simulink model "SolarPanelVarified"  (Simulink 7.5)
settings: Solver=ode45  StartTime=0.0  StopTime=10  RelTol=1e-3
undefined symbols (not defined in the file): Hydride, Metal, Nickel
libraries: elec_lib x72, fl_lib x4, nesl_utility x4, electricdrivelib x1, powerlib x1
settings Model: Creator=Satendra  LastModifiedBy=Satendra

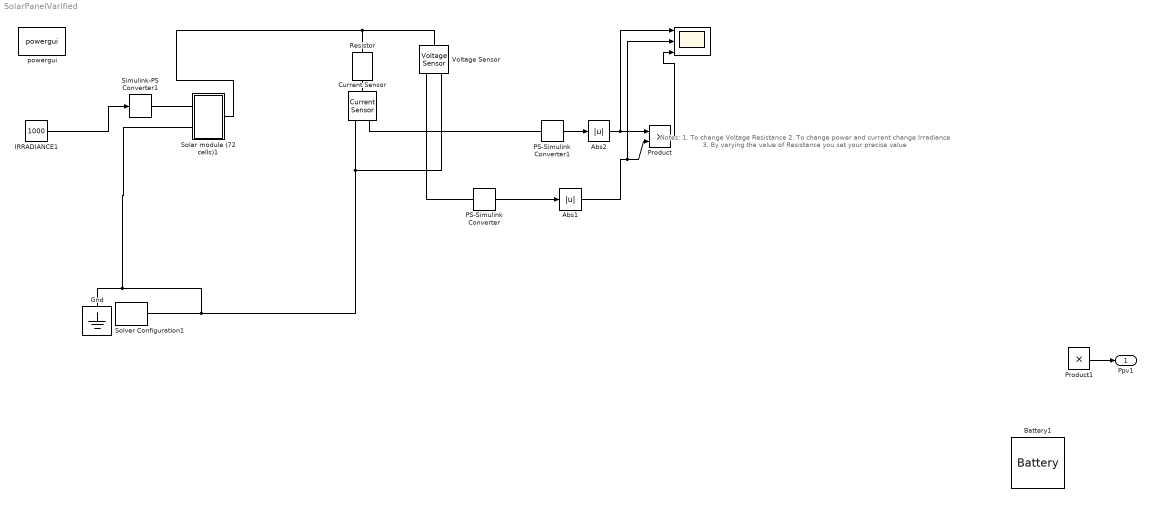
== system SolarPanelVarified ==
  note: Notes:
      | 1. To change Voltage Resistance
      | 2. To change power and current change Irradiance
      | 3. By varying the value of Resistance you set your precise value
  " " : Scope  NumInputPorts=3
      settings: TickLabels=on  YMin=-5~-5~-5  YMax=5~5~5
  Abs1 : Abs
  Abs2 : Abs
  Battery1 : electricdrivelib/Extra Sources/Battery  DialogController=POWERSYS.PowerSysDialog  SystemSampleTime=-1  BatType=Nickel-Metal-Hydride  ShowDetailedParameters=off  NomV=1.2  NomQ=1.5  SOC=100  PresetModel=on  MaxQ=1.6154  FullV=1.4136  Dis_rate=0.3  R=0.008  Normal_OP=1.4423  expZone="[1.3017         0.3]"  Dis_Char=off  current=[1.5 3]  Units=Ampere-hour  Batt_Tr=30
  Current Sensor : fl_lib/Electrical/Electrical Sensors/Current Sensor  DialogController=NetworkEngine.DynNeDlgSource  SystemSampleTime=-1  i1_Log=off  v1_Log=off  LocalVarNames=|i1|v1  LocalVarDescs=|i1|v1  LocalVarLogging=[0 0]
  Gnd : fl_lib/Electrical/Electrical Elements/Electrical Reference  DialogController=NetworkEngine.DynNeDlgSource  SystemSampleTime=-1  i_Log=off  LocalVarNames=|i  LocalVarDescs=|i  LocalVarLogging=[]
  IRRADIANCE1 : Constant  Value=1000
  PS-Simulink Converter : nesl_utility/PS-Simulink Converter  DialogController=NetworkEngine.DynNeUtilDlgSource  SystemSampleTime=-1  PhysicalDomain=network_engine_domain  LeftPortType=input  RightPortType=output  SubClassName=ps_output  Unit=1  AffineConversion=off
  PS-Simulink Converter1 : nesl_utility/PS-Simulink Converter  DialogController=NetworkEngine.DynNeUtilDlgSource  SystemSampleTime=-1  PhysicalDomain=network_engine_domain  LeftPortType=input  RightPortType=output  SubClassName=ps_output  Unit=1  AffineConversion=off
  Product : Product  RndMeth=Zero
  Product1 : Product  RndMeth=Zero
  Resistor : fl_lib/Electrical/Electrical Elements/Resistor  DialogController=NetworkEngine.DynNeDlgSource  SystemSampleTime=-1  R=3 Ohm  i_Log=off  v_Log=off  LocalVarNames=|i|v  LocalVarDescs=|i|v  LocalVarLogging=[0 0]
  Simulink-PS Converter1 : nesl_utility/Simulink-PS Converter  DialogController=NetworkEngine.DynNeUtilDlgSource  SystemSampleTime=-1  PhysicalDomain=network_engine_domain  LeftPortType=input  RightPortType=output  SubClassName=ps_input  Unit=1  AffineConversion=off  InputFilterTimeConstant=.001  UdotUserProvided=0
  Solar module (72 cells)1 : Subsystem
  Solver Configuration1 : nesl_utility/Solver Configuration  DialogController=NetworkEngine.DynNeUtilDlgSource  SystemSampleTime=-1  PhysicalDomain=network_engine_domain  LeftPortType=input  RightPortType=generic  SubClassName=solver  Accelerate=off  Profile=off  ResidualTolerance=1e-9  MaxNonlinIter=3  MaxModeIter=2  DoFixedCost=off  UseLocalSampling=off  DoDC=off  LinearAlgebra=Sparse  LocalSolverSampleTime=.001  LocalSolverChoice=NE_BACKWARD_EULER_ADVANCER  UseLocalSolver=off
  Voltage Sensor : fl_lib/Electrical/Electrical Sensors/Voltage Sensor  DialogController=NetworkEngine.DynNeDlgSource  SystemSampleTime=-1  i1_Log=off  v1_Log=off  LocalVarNames=|i1|v1  LocalVarDescs=|i1|v1  LocalVarLogging=[0 0]
  powergui : powerlib/powergui  Priority=1  SystemSampleTime=-1  SimulationMode=Continuous  SampleTime=50e-6  frequency=60  SPID=off  DisableSnubberDevices=off  DisableRonSwitches=off  DisableVfSwitches=off  SwTol=0  Interpol=off  frequencyindice=0  echomessages=off  HookPort=off  DisplayEquations=off  FunctionMessages=off  EnableUseOfTLC=off  x0status=blocks  RestoreLinks=warning  ResistiveCurrentMeasurement=off  Ylog=off  Xlog=on  ShowGrid=off  save=off  variable=ZData  ZoomFFT=off  StartTime=0.0  cycles=1  DisplayStyle=1  FreqAxis=off  MaxFrequency=1000  frequencyindicesteady=1  display=off  methode=off
  Ppv1 : Outport
  wires:
  PS-Simulink Converter1/1 -> Abs2/1
  PS-Simulink Converter/1 -> Abs1/1
  Abs1/1 -> Product/2, " "/2
  Abs2/1 -> Product/1, " "/1
  Product1/1 -> Ppv1/1
  Product/1 -> " "/3
  IRRADIANCE1/1 -> Simulink-PS Converter1/1
  connections:
  Current Sensor/RConn1 -- PS-Simulink Converter1/LConn1
  Solar module (72 cells)1/RConn1 -- Resistor/LConn1 -- Voltage Sensor/LConn1
  Resistor/RConn1 -- Current Sensor/LConn1
  Voltage Sensor/RConn1 -- PS-Simulink Converter/LConn1
  Solar module (72 cells)1/LConn2 -- Solver Configuration1/RConn1 -- Voltage Sensor/RConn2 -- Current Sensor/RConn2 -- Gnd/LConn1
  Simulink-PS Converter1/RConn1 -- Solar module (72 cells)1/LConn1

== system SolarPanelVarified/Solar module (72 cells)1 ==
  36 solarceel : Subsystem
  36 solarceel1 : Subsystem
  Ir : PMIOPort  Port=1  Side=Left
  + : PMIOPort  Port=2  Side=Right
  - : PMIOPort  Port=3  Side=Left
  connections:
  Ir/RConn1 -- 36 solarceel/LConn1 -- 36 solarceel1/LConn1
  36 solarceel/RConn1 -- 36 solarceel1/LConn2
  +/RConn1 -- 36 solarceel1/RConn1
  -/RConn1 -- 36 solarceel/LConn2

== system SolarPanelVarified/Solar module (72 cells)1/36 solarceel ==
  18 solar cells : Subsystem
  18 solar cells1 : Subsystem
  Ir : PMIOPort  Port=1  Side=Left
  + : PMIOPort  Port=2  Side=Right
  - : PMIOPort  Port=3  Side=Left
  connections:
  Ir/RConn1 -- 18 solar cells1/LConn1 -- 18 solar cells/LConn1
  18 solar cells/RConn1 -- 18 solar cells1/LConn2
  +/RConn1 -- 18 solar cells1/RConn1
  -/RConn1 -- 18 solar cells/LConn2

== system SolarPanelVarified/Solar module (72 cells)1/36 solarceel1 ==
  18 solar cells : Subsystem
  18 solar cells1 : Subsystem
  Ir : PMIOPort  Port=1  Side=Left
  + : PMIOPort  Port=2  Side=Right
  - : PMIOPort  Port=3  Side=Left
  connections:
  18 solar cells/LConn1 -- Ir/RConn1 -- 18 solar cells1/LConn1
  18 solar cells/RConn1 -- 18 solar cells1/LConn2
  +/RConn1 -- 18 solar cells1/RConn1
  -/RConn1 -- 18 solar cells/LConn2

== system SolarPanelVarified/Solar module (72 cells)1/36 solarceel/18 solar cells ==
  6solarcells : Subsystem
  6solarcells1 : Subsystem
  6solarcells2 : Subsystem
  + : PMIOPort  Port=1  Side=Right
  Ir : PMIOPort  Port=2  Side=Left
  - : PMIOPort  Port=3  Side=Left
  connections:
  Ir/RConn1 -- 6solarcells1/LConn1 -- 6solarcells/LConn1 -- 6solarcells2/LConn1
  6solarcells/RConn1 -- 6solarcells1/LConn2
  6solarcells1/RConn1 -- 6solarcells2/LConn2
  +/RConn1 -- 6solarcells2/RConn1
  -/RConn1 -- 6solarcells/LConn2

== system SolarPanelVarified/Solar module (72 cells)1/36 solarceel/18 solar cells1 ==
  6solarcells : Subsystem
  6solarcells1 : Subsystem
  6solarcells2 : Subsystem
  + : PMIOPort  Port=1  Side=Right
  Ir : PMIOPort  Port=2  Side=Left
  - : PMIOPort  Port=3  Side=Left
  connections:
  6solarcells1/LConn1 -- 6solarcells/LConn1 -- Ir/RConn1 -- 6solarcells2/LConn1
  6solarcells/RConn1 -- 6solarcells1/LConn2
  6solarcells1/RConn1 -- 6solarcells2/LConn2
  +/RConn1 -- 6solarcells2/RConn1
  -/RConn1 -- 6solarcells/LConn2

== system SolarPanelVarified/Solar module (72 cells)1/36 solarceel1/18 solar cells ==
  6solarcells : Subsystem
  6solarcells1 : Subsystem
  6solarcells2 : Subsystem
  + : PMIOPort  Port=1  Side=Right
  Ir : PMIOPort  Port=2  Side=Left
  - : PMIOPort  Port=3  Side=Left
  connections:
  6solarcells1/LConn1 -- 6solarcells/LConn1 -- Ir/RConn1 -- 6solarcells2/LConn1
  6solarcells/RConn1 -- 6solarcells1/LConn2
  6solarcells1/RConn1 -- 6solarcells2/LConn2
  +/RConn1 -- 6solarcells2/RConn1
  -/RConn1 -- 6solarcells/LConn2

== system SolarPanelVarified/Solar module (72 cells)1/36 solarceel1/18 solar cells1 ==
  6solarcells : Subsystem
  6solarcells1 : Subsystem
  6solarcells2 : Subsystem
  + : PMIOPort  Port=1  Side=Right
  Ir : PMIOPort  Port=2  Side=Left
  - : PMIOPort  Port=3  Side=Left
  connections:
  6solarcells1/LConn1 -- 6solarcells/LConn1 -- Ir/RConn1 -- 6solarcells2/LConn1
  6solarcells/RConn1 -- 6solarcells1/LConn2
  6solarcells1/RConn1 -- 6solarcells2/LConn2
  +/RConn1 -- 6solarcells2/RConn1
  -/RConn1 -- 6solarcells/LConn2

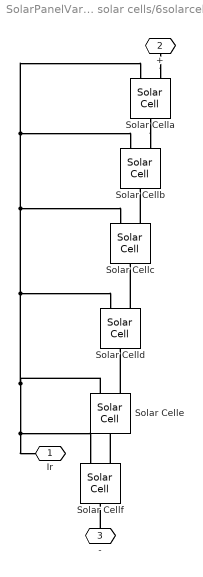
== system SolarPanelVarified/Solar module (72 cells)1/36 solarceel/18 solar cells/6solarcells ==
  Solar Cella : elec_lib/Sources/Solar Cell  DialogController=NetworkEngine.DynNeDlgSource  SystemSampleTime=-1  prm=1  Isc=4.75 A  Voc=0.6 V  Is=1e-6 A  Is2=0 A  Iph=7.34 A  Ir0=1000 W/m^2  ec=1.6  N2=2  Rs=5.1e-3 Ohm  Rp=Inf Ohm  TIPH1=0.65e-3 1/K  EG=1.12 eV  TXIS1=3  TXIS2=3  TRS1=0  TRP1=0  TFIXED=25 C  Tmeas=25 C  LocalVarLogging=[]
  Solar Cellb : elec_lib/Sources/Solar Cell  DialogController=NetworkEngine.DynNeDlgSource  SystemSampleTime=-1  prm=1  Isc=4.75 A  Voc=0.6 V  Is=1e-6 A  Is2=0 A  Iph=7.34 A  Ir0=1000 W/m^2  ec=1.6  N2=2  Rs=5.1e-3 Ohm  Rp=Inf Ohm  TIPH1=0.65e-3 1/K  EG=1.12 eV  TXIS1=3  TXIS2=3  TRS1=0  TRP1=0  TFIXED=25 C  Tmeas=25 C  LocalVarLogging=[]
  Solar Cellc : elec_lib/Sources/Solar Cell  DialogController=NetworkEngine.DynNeDlgSource  SystemSampleTime=-1  prm=1  Isc=4.75 A  Voc=0.6 V  Is=1e-6 A  Is2=0 A  Iph=7.34 A  Ir0=1000 W/m^2  ec=1.6  N2=2  Rs=5.1e-3 Ohm  Rp=Inf Ohm  TIPH1=0.65e-3 1/K  EG=1.12 eV  TXIS1=3  TXIS2=3  TRS1=0  TRP1=0  TFIXED=25 C  Tmeas=25 C  LocalVarLogging=[]
  Solar Celld : elec_lib/Sources/Solar Cell  DialogController=NetworkEngine.DynNeDlgSource  SystemSampleTime=-1  prm=1  Isc=4.75 A  Voc=0.6 V  Is=1e-6 A  Is2=0 A  Iph=7.34 A  Ir0=1000 W/m^2  ec=1.6  N2=2  Rs=5.1e-3 Ohm  Rp=Inf Ohm  TIPH1=0.65e-3 1/K  EG=1.12 eV  TXIS1=3  TXIS2=3  TRS1=0  TRP1=0  TFIXED=25 C  Tmeas=25 C  LocalVarLogging=[]
  Solar Celle : elec_lib/Sources/Solar Cell  DialogController=NetworkEngine.DynNeDlgSource  SystemSampleTime=-1  prm=1  Isc=4.75 A  Voc=0.6 V  Is=1e-6 A  Is2=0 A  Iph=7.34 A  Ir0=1000 W/m^2  ec=1.6  N2=2  Rs=5.1e-3 Ohm  Rp=Inf Ohm  TIPH1=0.65e-3 1/K  EG=1.12 eV  TXIS1=3  TXIS2=3  TRS1=0  TRP1=0  TFIXED=25 C  Tmeas=25 C  LocalVarLogging=[]
  Solar Cellf : elec_lib/Sources/Solar Cell  DialogController=NetworkEngine.DynNeDlgSource  SystemSampleTime=-1  prm=1  Isc=4.75 A  Voc=0.6 V  Is=1e-6 A  Is2=0 A  Iph=7.34 A  Ir0=1000 W/m^2  ec=1.6  N2=2  Rs=5.1e-3 Ohm  Rp=Inf Ohm  TIPH1=0.65e-3 1/K  EG=1.12 eV  TXIS1=3  TXIS2=3  TRS1=0  TRP1=0  TFIXED=25 C  Tmeas=25 C  LocalVarLogging=[]
  Ir : PMIOPort  Port=1  Side=Left
  + : PMIOPort  Port=2  Side=Right
  - : PMIOPort  Port=3  Side=Left
  connections:
  Ir/RConn1 -- Solar Celle/LConn1 -- Solar Celld/LConn1 -- Solar Cellc/LConn1 -- Solar Cellb/LConn1 -- Solar Cella/LConn1 -- Solar Cellf/LConn1
  Solar Cella/RConn1 -- Solar Cellb/LConn2
  Solar Cellc/LConn2 -- Solar Cellb/RConn1
  Solar Celld/LConn2 -- Solar Cellc/RConn1
  Solar Celle/LConn2 -- Solar Celld/RConn1
  Solar Cellf/LConn2 -- Solar Celle/RConn1
  +/RConn1 -- Solar Cella/LConn2
  -/RConn1 -- Solar Cellf/RConn1

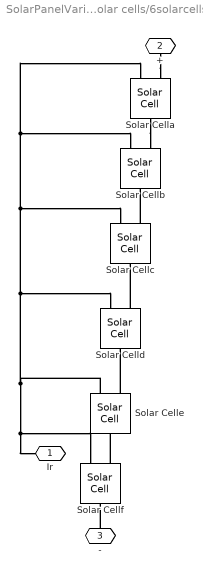
== system SolarPanelVarified/Solar module (72 cells)1/36 solarceel/18 solar cells/6solarcells1 ==
  Solar Cella : elec_lib/Sources/Solar Cell  DialogController=NetworkEngine.DynNeDlgSource  SystemSampleTime=-1  prm=1  Isc=4.75 A  Voc=0.6 V  Is=1e-6 A  Is2=0 A  Iph=7.34 A  Ir0=1000 W/m^2  ec=1.6  N2=2  Rs=5.1e-3 Ohm  Rp=Inf Ohm  TIPH1=0.65e-3 1/K  EG=1.12 eV  TXIS1=3  TXIS2=3  TRS1=0  TRP1=0  TFIXED=25 C  Tmeas=25 C  LocalVarLogging=[]
  Solar Cellb : elec_lib/Sources/Solar Cell  DialogController=NetworkEngine.DynNeDlgSource  SystemSampleTime=-1  prm=1  Isc=4.75 A  Voc=0.6 V  Is=1e-6 A  Is2=0 A  Iph=7.34 A  Ir0=1000 W/m^2  ec=1.6  N2=2  Rs=5.1e-3 Ohm  Rp=Inf Ohm  TIPH1=0.65e-3 1/K  EG=1.12 eV  TXIS1=3  TXIS2=3  TRS1=0  TRP1=0  TFIXED=25 C  Tmeas=25 C  LocalVarLogging=[]
  Solar Cellc : elec_lib/Sources/Solar Cell  DialogController=NetworkEngine.DynNeDlgSource  SystemSampleTime=-1  prm=1  Isc=4.75 A  Voc=0.6 V  Is=1e-6 A  Is2=0 A  Iph=7.34 A  Ir0=1000 W/m^2  ec=1.6  N2=2  Rs=5.1e-3 Ohm  Rp=Inf Ohm  TIPH1=0.65e-3 1/K  EG=1.12 eV  TXIS1=3  TXIS2=3  TRS1=0  TRP1=0  TFIXED=25 C  Tmeas=25 C  LocalVarLogging=[]
  Solar Celld : elec_lib/Sources/Solar Cell  DialogController=NetworkEngine.DynNeDlgSource  SystemSampleTime=-1  prm=1  Isc=4.75 A  Voc=0.6 V  Is=1e-6 A  Is2=0 A  Iph=7.34 A  Ir0=1000 W/m^2  ec=1.6  N2=2  Rs=5.1e-3 Ohm  Rp=Inf Ohm  TIPH1=0.65e-3 1/K  EG=1.12 eV  TXIS1=3  TXIS2=3  TRS1=0  TRP1=0  TFIXED=25 C  Tmeas=25 C  LocalVarLogging=[]
  Solar Celle : elec_lib/Sources/Solar Cell  DialogController=NetworkEngine.DynNeDlgSource  SystemSampleTime=-1  prm=1  Isc=4.75 A  Voc=0.6 V  Is=1e-6 A  Is2=0 A  Iph=7.34 A  Ir0=1000 W/m^2  ec=1.6  N2=2  Rs=5.1e-3 Ohm  Rp=Inf Ohm  TIPH1=0.65e-3 1/K  EG=1.12 eV  TXIS1=3  TXIS2=3  TRS1=0  TRP1=0  TFIXED=25 C  Tmeas=25 C  LocalVarLogging=[]
  Solar Cellf : elec_lib/Sources/Solar Cell  DialogController=NetworkEngine.DynNeDlgSource  SystemSampleTime=-1  prm=1  Isc=4.75 A  Voc=0.6 V  Is=1e-6 A  Is2=0 A  Iph=7.34 A  Ir0=1000 W/m^2  ec=1.6  N2=2  Rs=5.1e-3 Ohm  Rp=Inf Ohm  TIPH1=0.65e-3 1/K  EG=1.12 eV  TXIS1=3  TXIS2=3  TRS1=0  TRP1=0  TFIXED=25 C  Tmeas=25 C  LocalVarLogging=[]
  Ir : PMIOPort  Port=1  Side=Left
  + : PMIOPort  Port=2  Side=Right
  - : PMIOPort  Port=3  Side=Left
  connections:
  Solar Celle/LConn1 -- Solar Cellf/LConn1 -- Ir/RConn1 -- Solar Celld/LConn1 -- Solar Cellc/LConn1 -- Solar Cella/LConn1 -- Solar Cellb/LConn1
  Solar Cella/RConn1 -- Solar Cellb/LConn2
  Solar Cellc/LConn2 -- Solar Cellb/RConn1
  Solar Celld/LConn2 -- Solar Cellc/RConn1
  Solar Celle/LConn2 -- Solar Celld/RConn1
  Solar Cellf/LConn2 -- Solar Celle/RConn1
  +/RConn1 -- Solar Cella/LConn2
  -/RConn1 -- Solar Cellf/RConn1

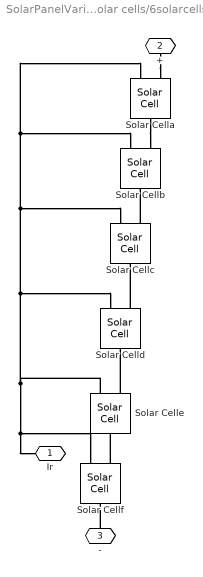
== system SolarPanelVarified/Solar module (72 cells)1/36 solarceel/18 solar cells/6solarcells2 ==
  Solar Cella : elec_lib/Sources/Solar Cell  DialogController=NetworkEngine.DynNeDlgSource  SystemSampleTime=-1  prm=1  Isc=4.75 A  Voc=0.6 V  Is=1e-6 A  Is2=0 A  Iph=7.34 A  Ir0=1000 W/m^2  ec=1.6  N2=2  Rs=5.1e-3 Ohm  Rp=Inf Ohm  TIPH1=0.65e-3 1/K  EG=1.12 eV  TXIS1=3  TXIS2=3  TRS1=0  TRP1=0  TFIXED=25 C  Tmeas=25 C  LocalVarLogging=[]
  Solar Cellb : elec_lib/Sources/Solar Cell  DialogController=NetworkEngine.DynNeDlgSource  SystemSampleTime=-1  prm=1  Isc=4.75 A  Voc=0.6 V  Is=1e-6 A  Is2=0 A  Iph=7.34 A  Ir0=1000 W/m^2  ec=1.6  N2=2  Rs=5.1e-3 Ohm  Rp=Inf Ohm  TIPH1=0.65e-3 1/K  EG=1.12 eV  TXIS1=3  TXIS2=3  TRS1=0  TRP1=0  TFIXED=25 C  Tmeas=25 C  LocalVarLogging=[]
  Solar Cellc : elec_lib/Sources/Solar Cell  DialogController=NetworkEngine.DynNeDlgSource  SystemSampleTime=-1  prm=1  Isc=4.75 A  Voc=0.6 V  Is=1e-6 A  Is2=0 A  Iph=7.34 A  Ir0=1000 W/m^2  ec=1.6  N2=2  Rs=5.1e-3 Ohm  Rp=Inf Ohm  TIPH1=0.65e-3 1/K  EG=1.12 eV  TXIS1=3  TXIS2=3  TRS1=0  TRP1=0  TFIXED=25 C  Tmeas=25 C  LocalVarLogging=[]
  Solar Celld : elec_lib/Sources/Solar Cell  DialogController=NetworkEngine.DynNeDlgSource  SystemSampleTime=-1  prm=1  Isc=4.75 A  Voc=0.6 V  Is=1e-6 A  Is2=0 A  Iph=7.34 A  Ir0=1000 W/m^2  ec=1.6  N2=2  Rs=5.1e-3 Ohm  Rp=Inf Ohm  TIPH1=0.65e-3 1/K  EG=1.12 eV  TXIS1=3  TXIS2=3  TRS1=0  TRP1=0  TFIXED=25 C  Tmeas=25 C  LocalVarLogging=[]
  Solar Celle : elec_lib/Sources/Solar Cell  DialogController=NetworkEngine.DynNeDlgSource  SystemSampleTime=-1  prm=1  Isc=4.75 A  Voc=0.6 V  Is=1e-6 A  Is2=0 A  Iph=7.34 A  Ir0=1000 W/m^2  ec=1.6  N2=2  Rs=5.1e-3 Ohm  Rp=Inf Ohm  TIPH1=0.65e-3 1/K  EG=1.12 eV  TXIS1=3  TXIS2=3  TRS1=0  TRP1=0  TFIXED=25 C  Tmeas=25 C  LocalVarLogging=[]
  Solar Cellf : elec_lib/Sources/Solar Cell  DialogController=NetworkEngine.DynNeDlgSource  SystemSampleTime=-1  prm=1  Isc=4.75 A  Voc=0.6 V  Is=1e-6 A  Is2=0 A  Iph=7.34 A  Ir0=1000 W/m^2  ec=1.6  N2=2  Rs=5.1e-3 Ohm  Rp=Inf Ohm  TIPH1=0.65e-3 1/K  EG=1.12 eV  TXIS1=3  TXIS2=3  TRS1=0  TRP1=0  TFIXED=25 C  Tmeas=25 C  LocalVarLogging=[]
  Ir : PMIOPort  Port=1  Side=Left
  + : PMIOPort  Port=2  Side=Right
  - : PMIOPort  Port=3  Side=Left
  connections:
  Solar Celle/LConn1 -- Solar Cellf/LConn1 -- Ir/RConn1 -- Solar Celld/LConn1 -- Solar Cellc/LConn1 -- Solar Cella/LConn1 -- Solar Cellb/LConn1
  Solar Cella/RConn1 -- Solar Cellb/LConn2
  Solar Cellc/LConn2 -- Solar Cellb/RConn1
  Solar Celld/LConn2 -- Solar Cellc/RConn1
  Solar Celle/LConn2 -- Solar Celld/RConn1
  Solar Cellf/LConn2 -- Solar Celle/RConn1
  +/RConn1 -- Solar Cella/LConn2
  -/RConn1 -- Solar Cellf/RConn1

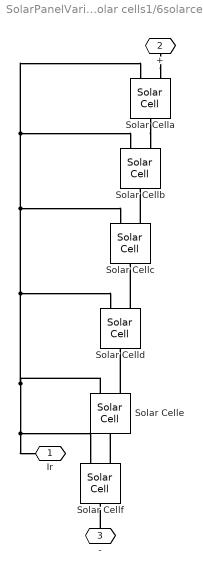
== system SolarPanelVarified/Solar module (72 cells)1/36 solarceel/18 solar cells1/6solarcells ==
  Solar Cella : elec_lib/Sources/Solar Cell  DialogController=NetworkEngine.DynNeDlgSource  SystemSampleTime=-1  prm=1  Isc=4.75 A  Voc=0.6 V  Is=1e-6 A  Is2=0 A  Iph=7.34 A  Ir0=1000 W/m^2  ec=1.6  N2=2  Rs=5.1e-3 Ohm  Rp=Inf Ohm  TIPH1=0.65e-3 1/K  EG=1.12 eV  TXIS1=3  TXIS2=3  TRS1=0  TRP1=0  TFIXED=25 C  Tmeas=25 C  LocalVarLogging=[]
  Solar Cellb : elec_lib/Sources/Solar Cell  DialogController=NetworkEngine.DynNeDlgSource  SystemSampleTime=-1  prm=1  Isc=4.75 A  Voc=0.6 V  Is=1e-6 A  Is2=0 A  Iph=7.34 A  Ir0=1000 W/m^2  ec=1.6  N2=2  Rs=5.1e-3 Ohm  Rp=Inf Ohm  TIPH1=0.65e-3 1/K  EG=1.12 eV  TXIS1=3  TXIS2=3  TRS1=0  TRP1=0  TFIXED=25 C  Tmeas=25 C  LocalVarLogging=[]
  Solar Cellc : elec_lib/Sources/Solar Cell  DialogController=NetworkEngine.DynNeDlgSource  SystemSampleTime=-1  prm=1  Isc=4.75 A  Voc=0.6 V  Is=1e-6 A  Is2=0 A  Iph=7.34 A  Ir0=1000 W/m^2  ec=1.6  N2=2  Rs=5.1e-3 Ohm  Rp=Inf Ohm  TIPH1=0.65e-3 1/K  EG=1.12 eV  TXIS1=3  TXIS2=3  TRS1=0  TRP1=0  TFIXED=25 C  Tmeas=25 C  LocalVarLogging=[]
  Solar Celld : elec_lib/Sources/Solar Cell  DialogController=NetworkEngine.DynNeDlgSource  SystemSampleTime=-1  prm=1  Isc=4.75 A  Voc=0.6 V  Is=1e-6 A  Is2=0 A  Iph=7.34 A  Ir0=1000 W/m^2  ec=1.6  N2=2  Rs=5.1e-3 Ohm  Rp=Inf Ohm  TIPH1=0.65e-3 1/K  EG=1.12 eV  TXIS1=3  TXIS2=3  TRS1=0  TRP1=0  TFIXED=25 C  Tmeas=25 C  LocalVarLogging=[]
  Solar Celle : elec_lib/Sources/Solar Cell  DialogController=NetworkEngine.DynNeDlgSource  SystemSampleTime=-1  prm=1  Isc=4.75 A  Voc=0.6 V  Is=1e-6 A  Is2=0 A  Iph=7.34 A  Ir0=1000 W/m^2  ec=1.6  N2=2  Rs=5.1e-3 Ohm  Rp=Inf Ohm  TIPH1=0.65e-3 1/K  EG=1.12 eV  TXIS1=3  TXIS2=3  TRS1=0  TRP1=0  TFIXED=25 C  Tmeas=25 C  LocalVarLogging=[]
  Solar Cellf : elec_lib/Sources/Solar Cell  DialogController=NetworkEngine.DynNeDlgSource  SystemSampleTime=-1  prm=1  Isc=4.75 A  Voc=0.6 V  Is=1e-6 A  Is2=0 A  Iph=7.34 A  Ir0=1000 W/m^2  ec=1.6  N2=2  Rs=5.1e-3 Ohm  Rp=Inf Ohm  TIPH1=0.65e-3 1/K  EG=1.12 eV  TXIS1=3  TXIS2=3  TRS1=0  TRP1=0  TFIXED=25 C  Tmeas=25 C  LocalVarLogging=[]
  Ir : PMIOPort  Port=1  Side=Left
  + : PMIOPort  Port=2  Side=Right
  - : PMIOPort  Port=3  Side=Left
  connections:
  Solar Celle/LConn1 -- Solar Cellf/LConn1 -- Ir/RConn1 -- Solar Celld/LConn1 -- Solar Cellc/LConn1 -- Solar Cella/LConn1 -- Solar Cellb/LConn1
  Solar Cella/RConn1 -- Solar Cellb/LConn2
  Solar Cellc/LConn2 -- Solar Cellb/RConn1
  Solar Celld/LConn2 -- Solar Cellc/RConn1
  Solar Celle/LConn2 -- Solar Celld/RConn1
  Solar Cellf/LConn2 -- Solar Celle/RConn1
  +/RConn1 -- Solar Cella/LConn2
  -/RConn1 -- Solar Cellf/RConn1

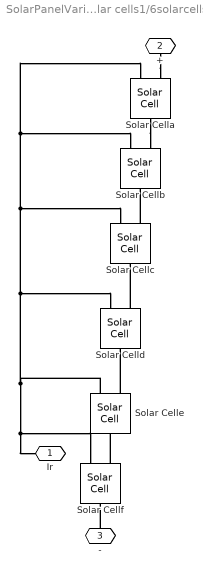
== system SolarPanelVarified/Solar module (72 cells)1/36 solarceel/18 solar cells1/6solarcells1 ==
  Solar Cella : elec_lib/Sources/Solar Cell  DialogController=NetworkEngine.DynNeDlgSource  SystemSampleTime=-1  prm=1  Isc=4.75 A  Voc=0.6 V  Is=1e-6 A  Is2=0 A  Iph=7.34 A  Ir0=1000 W/m^2  ec=1.6  N2=2  Rs=5.1e-3 Ohm  Rp=Inf Ohm  TIPH1=0.65e-3 1/K  EG=1.12 eV  TXIS1=3  TXIS2=3  TRS1=0  TRP1=0  TFIXED=25 C  Tmeas=25 C  LocalVarLogging=[]
  Solar Cellb : elec_lib/Sources/Solar Cell  DialogController=NetworkEngine.DynNeDlgSource  SystemSampleTime=-1  prm=1  Isc=4.75 A  Voc=0.6 V  Is=1e-6 A  Is2=0 A  Iph=7.34 A  Ir0=1000 W/m^2  ec=1.6  N2=2  Rs=5.1e-3 Ohm  Rp=Inf Ohm  TIPH1=0.65e-3 1/K  EG=1.12 eV  TXIS1=3  TXIS2=3  TRS1=0  TRP1=0  TFIXED=25 C  Tmeas=25 C  LocalVarLogging=[]
  Solar Cellc : elec_lib/Sources/Solar Cell  DialogController=NetworkEngine.DynNeDlgSource  SystemSampleTime=-1  prm=1  Isc=4.75 A  Voc=0.6 V  Is=1e-6 A  Is2=0 A  Iph=7.34 A  Ir0=1000 W/m^2  ec=1.6  N2=2  Rs=5.1e-3 Ohm  Rp=Inf Ohm  TIPH1=0.65e-3 1/K  EG=1.12 eV  TXIS1=3  TXIS2=3  TRS1=0  TRP1=0  TFIXED=25 C  Tmeas=25 C  LocalVarLogging=[]
  Solar Celld : elec_lib/Sources/Solar Cell  DialogController=NetworkEngine.DynNeDlgSource  SystemSampleTime=-1  prm=1  Isc=4.75 A  Voc=0.6 V  Is=1e-6 A  Is2=0 A  Iph=7.34 A  Ir0=1000 W/m^2  ec=1.6  N2=2  Rs=5.1e-3 Ohm  Rp=Inf Ohm  TIPH1=0.65e-3 1/K  EG=1.12 eV  TXIS1=3  TXIS2=3  TRS1=0  TRP1=0  TFIXED=25 C  Tmeas=25 C  LocalVarLogging=[]
  Solar Celle : elec_lib/Sources/Solar Cell  DialogController=NetworkEngine.DynNeDlgSource  SystemSampleTime=-1  prm=1  Isc=4.75 A  Voc=0.6 V  Is=1e-6 A  Is2=0 A  Iph=7.34 A  Ir0=1000 W/m^2  ec=1.6  N2=2  Rs=5.1e-3 Ohm  Rp=Inf Ohm  TIPH1=0.65e-3 1/K  EG=1.12 eV  TXIS1=3  TXIS2=3  TRS1=0  TRP1=0  TFIXED=25 C  Tmeas=25 C  LocalVarLogging=[]
  Solar Cellf : elec_lib/Sources/Solar Cell  DialogController=NetworkEngine.DynNeDlgSource  SystemSampleTime=-1  prm=1  Isc=4.75 A  Voc=0.6 V  Is=1e-6 A  Is2=0 A  Iph=7.34 A  Ir0=1000 W/m^2  ec=1.6  N2=2  Rs=5.1e-3 Ohm  Rp=Inf Ohm  TIPH1=0.65e-3 1/K  EG=1.12 eV  TXIS1=3  TXIS2=3  TRS1=0  TRP1=0  TFIXED=25 C  Tmeas=25 C  LocalVarLogging=[]
  Ir : PMIOPort  Port=1  Side=Left
  + : PMIOPort  Port=2  Side=Right
  - : PMIOPort  Port=3  Side=Left
  connections:
  Solar Celle/LConn1 -- Solar Cellf/LConn1 -- Ir/RConn1 -- Solar Celld/LConn1 -- Solar Cellc/LConn1 -- Solar Cella/LConn1 -- Solar Cellb/LConn1
  Solar Cella/RConn1 -- Solar Cellb/LConn2
  Solar Cellc/LConn2 -- Solar Cellb/RConn1
  Solar Celld/LConn2 -- Solar Cellc/RConn1
  Solar Celle/LConn2 -- Solar Celld/RConn1
  Solar Cellf/LConn2 -- Solar Celle/RConn1
  +/RConn1 -- Solar Cella/LConn2
  -/RConn1 -- Solar Cellf/RConn1

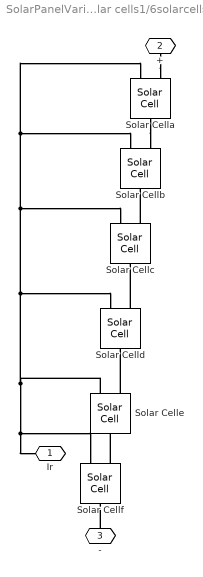
== system SolarPanelVarified/Solar module (72 cells)1/36 solarceel/18 solar cells1/6solarcells2 ==
  Solar Cella : elec_lib/Sources/Solar Cell  DialogController=NetworkEngine.DynNeDlgSource  SystemSampleTime=-1  prm=1  Isc=4.75 A  Voc=0.6 V  Is=1e-6 A  Is2=0 A  Iph=7.34 A  Ir0=1000 W/m^2  ec=1.6  N2=2  Rs=5.1e-3 Ohm  Rp=Inf Ohm  TIPH1=0.65e-3 1/K  EG=1.12 eV  TXIS1=3  TXIS2=3  TRS1=0  TRP1=0  TFIXED=25 C  Tmeas=25 C  LocalVarLogging=[]
  Solar Cellb : elec_lib/Sources/Solar Cell  DialogController=NetworkEngine.DynNeDlgSource  SystemSampleTime=-1  prm=1  Isc=4.75 A  Voc=0.6 V  Is=1e-6 A  Is2=0 A  Iph=7.34 A  Ir0=1000 W/m^2  ec=1.6  N2=2  Rs=5.1e-3 Ohm  Rp=Inf Ohm  TIPH1=0.65e-3 1/K  EG=1.12 eV  TXIS1=3  TXIS2=3  TRS1=0  TRP1=0  TFIXED=25 C  Tmeas=25 C  LocalVarLogging=[]
  Solar Cellc : elec_lib/Sources/Solar Cell  DialogController=NetworkEngine.DynNeDlgSource  SystemSampleTime=-1  prm=1  Isc=4.75 A  Voc=0.6 V  Is=1e-6 A  Is2=0 A  Iph=7.34 A  Ir0=1000 W/m^2  ec=1.6  N2=2  Rs=5.1e-3 Ohm  Rp=Inf Ohm  TIPH1=0.65e-3 1/K  EG=1.12 eV  TXIS1=3  TXIS2=3  TRS1=0  TRP1=0  TFIXED=25 C  Tmeas=25 C  LocalVarLogging=[]
  Solar Celld : elec_lib/Sources/Solar Cell  DialogController=NetworkEngine.DynNeDlgSource  SystemSampleTime=-1  prm=1  Isc=4.75 A  Voc=0.6 V  Is=1e-6 A  Is2=0 A  Iph=7.34 A  Ir0=1000 W/m^2  ec=1.6  N2=2  Rs=5.1e-3 Ohm  Rp=Inf Ohm  TIPH1=0.65e-3 1/K  EG=1.12 eV  TXIS1=3  TXIS2=3  TRS1=0  TRP1=0  TFIXED=25 C  Tmeas=25 C  LocalVarLogging=[]
  Solar Celle : elec_lib/Sources/Solar Cell  DialogController=NetworkEngine.DynNeDlgSource  SystemSampleTime=-1  prm=1  Isc=4.75 A  Voc=0.6 V  Is=1e-6 A  Is2=0 A  Iph=7.34 A  Ir0=1000 W/m^2  ec=1.6  N2=2  Rs=5.1e-3 Ohm  Rp=Inf Ohm  TIPH1=0.65e-3 1/K  EG=1.12 eV  TXIS1=3  TXIS2=3  TRS1=0  TRP1=0  TFIXED=25 C  Tmeas=25 C  LocalVarLogging=[]
  Solar Cellf : elec_lib/Sources/Solar Cell  DialogController=NetworkEngine.DynNeDlgSource  SystemSampleTime=-1  prm=1  Isc=4.75 A  Voc=0.6 V  Is=1e-6 A  Is2=0 A  Iph=7.34 A  Ir0=1000 W/m^2  ec=1.6  N2=2  Rs=5.1e-3 Ohm  Rp=Inf Ohm  TIPH1=0.65e-3 1/K  EG=1.12 eV  TXIS1=3  TXIS2=3  TRS1=0  TRP1=0  TFIXED=25 C  Tmeas=25 C  LocalVarLogging=[]
  Ir : PMIOPort  Port=1  Side=Left
  + : PMIOPort  Port=2  Side=Right
  - : PMIOPort  Port=3  Side=Left
  connections:
  Solar Celle/LConn1 -- Solar Cellf/LConn1 -- Ir/RConn1 -- Solar Celld/LConn1 -- Solar Cellc/LConn1 -- Solar Cella/LConn1 -- Solar Cellb/LConn1
  Solar Cella/RConn1 -- Solar Cellb/LConn2
  Solar Cellc/LConn2 -- Solar Cellb/RConn1
  Solar Celld/LConn2 -- Solar Cellc/RConn1
  Solar Celle/LConn2 -- Solar Celld/RConn1
  Solar Cellf/LConn2 -- Solar Celle/RConn1
  +/RConn1 -- Solar Cella/LConn2
  -/RConn1 -- Solar Cellf/RConn1

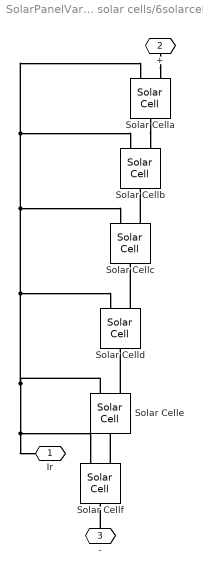
== system SolarPanelVarified/Solar module (72 cells)1/36 solarceel1/18 solar cells/6solarcells ==
  Solar Cella : elec_lib/Sources/Solar Cell  DialogController=NetworkEngine.DynNeDlgSource  SystemSampleTime=-1  prm=1  Isc=4.75 A  Voc=0.6 V  Is=1e-6 A  Is2=0 A  Iph=7.34 A  Ir0=1000 W/m^2  ec=1.6  N2=2  Rs=5.1e-3 Ohm  Rp=Inf Ohm  TIPH1=0.65e-3 1/K  EG=1.12 eV  TXIS1=3  TXIS2=3  TRS1=0  TRP1=0  TFIXED=25 C  Tmeas=25 C  LocalVarLogging=[]
  Solar Cellb : elec_lib/Sources/Solar Cell  DialogController=NetworkEngine.DynNeDlgSource  SystemSampleTime=-1  prm=1  Isc=4.75 A  Voc=0.6 V  Is=1e-6 A  Is2=0 A  Iph=7.34 A  Ir0=1000 W/m^2  ec=1.6  N2=2  Rs=5.1e-3 Ohm  Rp=Inf Ohm  TIPH1=0.65e-3 1/K  EG=1.12 eV  TXIS1=3  TXIS2=3  TRS1=0  TRP1=0  TFIXED=25 C  Tmeas=25 C  LocalVarLogging=[]
  Solar Cellc : elec_lib/Sources/Solar Cell  DialogController=NetworkEngine.DynNeDlgSource  SystemSampleTime=-1  prm=1  Isc=4.75 A  Voc=0.6 V  Is=1e-6 A  Is2=0 A  Iph=7.34 A  Ir0=1000 W/m^2  ec=1.6  N2=2  Rs=5.1e-3 Ohm  Rp=Inf Ohm  TIPH1=0.65e-3 1/K  EG=1.12 eV  TXIS1=3  TXIS2=3  TRS1=0  TRP1=0  TFIXED=25 C  Tmeas=25 C  LocalVarLogging=[]
  Solar Celld : elec_lib/Sources/Solar Cell  DialogController=NetworkEngine.DynNeDlgSource  SystemSampleTime=-1  prm=1  Isc=4.75 A  Voc=0.6 V  Is=1e-6 A  Is2=0 A  Iph=7.34 A  Ir0=1000 W/m^2  ec=1.6  N2=2  Rs=5.1e-3 Ohm  Rp=Inf Ohm  TIPH1=0.65e-3 1/K  EG=1.12 eV  TXIS1=3  TXIS2=3  TRS1=0  TRP1=0  TFIXED=25 C  Tmeas=25 C  LocalVarLogging=[]
  Solar Celle : elec_lib/Sources/Solar Cell  DialogController=NetworkEngine.DynNeDlgSource  SystemSampleTime=-1  prm=1  Isc=4.75 A  Voc=0.6 V  Is=1e-6 A  Is2=0 A  Iph=7.34 A  Ir0=1000 W/m^2  ec=1.6  N2=2  Rs=5.1e-3 Ohm  Rp=Inf Ohm  TIPH1=0.65e-3 1/K  EG=1.12 eV  TXIS1=3  TXIS2=3  TRS1=0  TRP1=0  TFIXED=25 C  Tmeas=25 C  LocalVarLogging=[]
  Solar Cellf : elec_lib/Sources/Solar Cell  DialogController=NetworkEngine.DynNeDlgSource  SystemSampleTime=-1  prm=1  Isc=4.75 A  Voc=0.6 V  Is=1e-6 A  Is2=0 A  Iph=7.34 A  Ir0=1000 W/m^2  ec=1.6  N2=2  Rs=5.1e-3 Ohm  Rp=Inf Ohm  TIPH1=0.65e-3 1/K  EG=1.12 eV  TXIS1=3  TXIS2=3  TRS1=0  TRP1=0  TFIXED=25 C  Tmeas=25 C  LocalVarLogging=[]
  Ir : PMIOPort  Port=1  Side=Left
  + : PMIOPort  Port=2  Side=Right
  - : PMIOPort  Port=3  Side=Left
  connections:
  Solar Celle/LConn1 -- Solar Cellf/LConn1 -- Ir/RConn1 -- Solar Celld/LConn1 -- Solar Cellc/LConn1 -- Solar Cella/LConn1 -- Solar Cellb/LConn1
  Solar Cella/RConn1 -- Solar Cellb/LConn2
  Solar Cellc/LConn2 -- Solar Cellb/RConn1
  Solar Celld/LConn2 -- Solar Cellc/RConn1
  Solar Celle/LConn2 -- Solar Celld/RConn1
  Solar Cellf/LConn2 -- Solar Celle/RConn1
  +/RConn1 -- Solar Cella/LConn2
  -/RConn1 -- Solar Cellf/RConn1

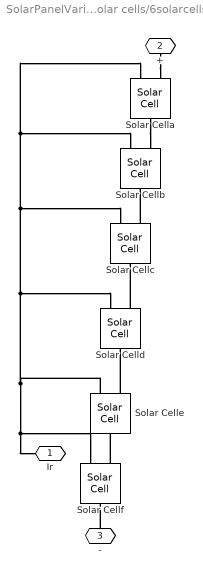
== system SolarPanelVarified/Solar module (72 cells)1/36 solarceel1/18 solar cells/6solarcells1 ==
  Solar Cella : elec_lib/Sources/Solar Cell  DialogController=NetworkEngine.DynNeDlgSource  SystemSampleTime=-1  prm=1  Isc=4.75 A  Voc=0.6 V  Is=1e-6 A  Is2=0 A  Iph=7.34 A  Ir0=1000 W/m^2  ec=1.6  N2=2  Rs=5.1e-3 Ohm  Rp=Inf Ohm  TIPH1=0.65e-3 1/K  EG=1.12 eV  TXIS1=3  TXIS2=3  TRS1=0  TRP1=0  TFIXED=25 C  Tmeas=25 C  LocalVarLogging=[]
  Solar Cellb : elec_lib/Sources/Solar Cell  DialogController=NetworkEngine.DynNeDlgSource  SystemSampleTime=-1  prm=1  Isc=4.75 A  Voc=0.6 V  Is=1e-6 A  Is2=0 A  Iph=7.34 A  Ir0=1000 W/m^2  ec=1.6  N2=2  Rs=5.1e-3 Ohm  Rp=Inf Ohm  TIPH1=0.65e-3 1/K  EG=1.12 eV  TXIS1=3  TXIS2=3  TRS1=0  TRP1=0  TFIXED=25 C  Tmeas=25 C  LocalVarLogging=[]
  Solar Cellc : elec_lib/Sources/Solar Cell  DialogController=NetworkEngine.DynNeDlgSource  SystemSampleTime=-1  prm=1  Isc=4.75 A  Voc=0.6 V  Is=1e-6 A  Is2=0 A  Iph=7.34 A  Ir0=1000 W/m^2  ec=1.6  N2=2  Rs=5.1e-3 Ohm  Rp=Inf Ohm  TIPH1=0.65e-3 1/K  EG=1.12 eV  TXIS1=3  TXIS2=3  TRS1=0  TRP1=0  TFIXED=25 C  Tmeas=25 C  LocalVarLogging=[]
  Solar Celld : elec_lib/Sources/Solar Cell  DialogController=NetworkEngine.DynNeDlgSource  SystemSampleTime=-1  prm=1  Isc=4.75 A  Voc=0.6 V  Is=1e-6 A  Is2=0 A  Iph=7.34 A  Ir0=1000 W/m^2  ec=1.6  N2=2  Rs=5.1e-3 Ohm  Rp=Inf Ohm  TIPH1=0.65e-3 1/K  EG=1.12 eV  TXIS1=3  TXIS2=3  TRS1=0  TRP1=0  TFIXED=25 C  Tmeas=25 C  LocalVarLogging=[]
  Solar Celle : elec_lib/Sources/Solar Cell  DialogController=NetworkEngine.DynNeDlgSource  SystemSampleTime=-1  prm=1  Isc=4.75 A  Voc=0.6 V  Is=1e-6 A  Is2=0 A  Iph=7.34 A  Ir0=1000 W/m^2  ec=1.6  N2=2  Rs=5.1e-3 Ohm  Rp=Inf Ohm  TIPH1=0.65e-3 1/K  EG=1.12 eV  TXIS1=3  TXIS2=3  TRS1=0  TRP1=0  TFIXED=25 C  Tmeas=25 C  LocalVarLogging=[]
  Solar Cellf : elec_lib/Sources/Solar Cell  DialogController=NetworkEngine.DynNeDlgSource  SystemSampleTime=-1  prm=1  Isc=4.75 A  Voc=0.6 V  Is=1e-6 A  Is2=0 A  Iph=7.34 A  Ir0=1000 W/m^2  ec=1.6  N2=2  Rs=5.1e-3 Ohm  Rp=Inf Ohm  TIPH1=0.65e-3 1/K  EG=1.12 eV  TXIS1=3  TXIS2=3  TRS1=0  TRP1=0  TFIXED=25 C  Tmeas=25 C  LocalVarLogging=[]
  Ir : PMIOPort  Port=1  Side=Left
  + : PMIOPort  Port=2  Side=Right
  - : PMIOPort  Port=3  Side=Left
  connections:
  Solar Celle/LConn1 -- Solar Cellf/LConn1 -- Ir/RConn1 -- Solar Celld/LConn1 -- Solar Cellc/LConn1 -- Solar Cella/LConn1 -- Solar Cellb/LConn1
  Solar Cella/RConn1 -- Solar Cellb/LConn2
  Solar Cellc/LConn2 -- Solar Cellb/RConn1
  Solar Celld/LConn2 -- Solar Cellc/RConn1
  Solar Celle/LConn2 -- Solar Celld/RConn1
  Solar Cellf/LConn2 -- Solar Celle/RConn1
  +/RConn1 -- Solar Cella/LConn2
  -/RConn1 -- Solar Cellf/RConn1

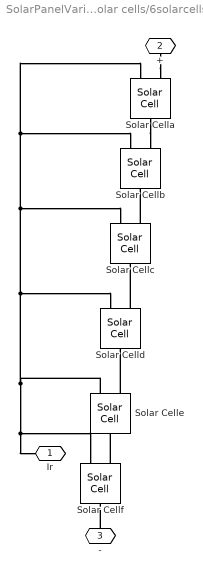
== system SolarPanelVarified/Solar module (72 cells)1/36 solarceel1/18 solar cells/6solarcells2 ==
  Solar Cella : elec_lib/Sources/Solar Cell  DialogController=NetworkEngine.DynNeDlgSource  SystemSampleTime=-1  prm=1  Isc=4.75 A  Voc=0.6 V  Is=1e-6 A  Is2=0 A  Iph=7.34 A  Ir0=1000 W/m^2  ec=1.6  N2=2  Rs=5.1e-3 Ohm  Rp=Inf Ohm  TIPH1=0.65e-3 1/K  EG=1.12 eV  TXIS1=3  TXIS2=3  TRS1=0  TRP1=0  TFIXED=25 C  Tmeas=25 C  LocalVarLogging=[]
  Solar Cellb : elec_lib/Sources/Solar Cell  DialogController=NetworkEngine.DynNeDlgSource  SystemSampleTime=-1  prm=1  Isc=4.75 A  Voc=0.6 V  Is=1e-6 A  Is2=0 A  Iph=7.34 A  Ir0=1000 W/m^2  ec=1.6  N2=2  Rs=5.1e-3 Ohm  Rp=Inf Ohm  TIPH1=0.65e-3 1/K  EG=1.12 eV  TXIS1=3  TXIS2=3  TRS1=0  TRP1=0  TFIXED=25 C  Tmeas=25 C  LocalVarLogging=[]
  Solar Cellc : elec_lib/Sources/Solar Cell  DialogController=NetworkEngine.DynNeDlgSource  SystemSampleTime=-1  prm=1  Isc=4.75 A  Voc=0.6 V  Is=1e-6 A  Is2=0 A  Iph=7.34 A  Ir0=1000 W/m^2  ec=1.6  N2=2  Rs=5.1e-3 Ohm  Rp=Inf Ohm  TIPH1=0.65e-3 1/K  EG=1.12 eV  TXIS1=3  TXIS2=3  TRS1=0  TRP1=0  TFIXED=25 C  Tmeas=25 C  LocalVarLogging=[]
  Solar Celld : elec_lib/Sources/Solar Cell  DialogController=NetworkEngine.DynNeDlgSource  SystemSampleTime=-1  prm=1  Isc=4.75 A  Voc=0.6 V  Is=1e-6 A  Is2=0 A  Iph=7.34 A  Ir0=1000 W/m^2  ec=1.6  N2=2  Rs=5.1e-3 Ohm  Rp=Inf Ohm  TIPH1=0.65e-3 1/K  EG=1.12 eV  TXIS1=3  TXIS2=3  TRS1=0  TRP1=0  TFIXED=25 C  Tmeas=25 C  LocalVarLogging=[]
  Solar Celle : elec_lib/Sources/Solar Cell  DialogController=NetworkEngine.DynNeDlgSource  SystemSampleTime=-1  prm=1  Isc=4.75 A  Voc=0.6 V  Is=1e-6 A  Is2=0 A  Iph=7.34 A  Ir0=1000 W/m^2  ec=1.6  N2=2  Rs=5.1e-3 Ohm  Rp=Inf Ohm  TIPH1=0.65e-3 1/K  EG=1.12 eV  TXIS1=3  TXIS2=3  TRS1=0  TRP1=0  TFIXED=25 C  Tmeas=25 C  LocalVarLogging=[]
  Solar Cellf : elec_lib/Sources/Solar Cell  DialogController=NetworkEngine.DynNeDlgSource  SystemSampleTime=-1  prm=1  Isc=4.75 A  Voc=0.6 V  Is=1e-6 A  Is2=0 A  Iph=7.34 A  Ir0=1000 W/m^2  ec=1.6  N2=2  Rs=5.1e-3 Ohm  Rp=Inf Ohm  TIPH1=0.65e-3 1/K  EG=1.12 eV  TXIS1=3  TXIS2=3  TRS1=0  TRP1=0  TFIXED=25 C  Tmeas=25 C  LocalVarLogging=[]
  Ir : PMIOPort  Port=1  Side=Left
  + : PMIOPort  Port=2  Side=Right
  - : PMIOPort  Port=3  Side=Left
  connections:
  Solar Celle/LConn1 -- Solar Cellf/LConn1 -- Ir/RConn1 -- Solar Celld/LConn1 -- Solar Cellc/LConn1 -- Solar Cella/LConn1 -- Solar Cellb/LConn1
  Solar Cella/RConn1 -- Solar Cellb/LConn2
  Solar Cellc/LConn2 -- Solar Cellb/RConn1
  Solar Celld/LConn2 -- Solar Cellc/RConn1
  Solar Celle/LConn2 -- Solar Celld/RConn1
  Solar Cellf/LConn2 -- Solar Celle/RConn1
  +/RConn1 -- Solar Cella/LConn2
  -/RConn1 -- Solar Cellf/RConn1

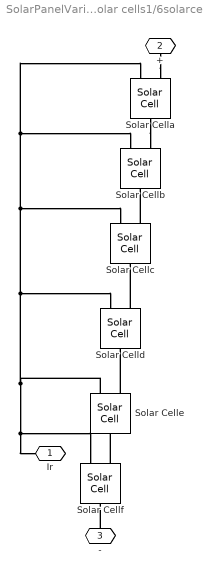
== system SolarPanelVarified/Solar module (72 cells)1/36 solarceel1/18 solar cells1/6solarcells ==
  Solar Cella : elec_lib/Sources/Solar Cell  DialogController=NetworkEngine.DynNeDlgSource  SystemSampleTime=-1  prm=1  Isc=4.75 A  Voc=0.6 V  Is=1e-6 A  Is2=0 A  Iph=7.34 A  Ir0=1000 W/m^2  ec=1.6  N2=2  Rs=5.1e-3 Ohm  Rp=Inf Ohm  TIPH1=0.65e-3 1/K  EG=1.12 eV  TXIS1=3  TXIS2=3  TRS1=0  TRP1=0  TFIXED=25 C  Tmeas=25 C  LocalVarLogging=[]
  Solar Cellb : elec_lib/Sources/Solar Cell  DialogController=NetworkEngine.DynNeDlgSource  SystemSampleTime=-1  prm=1  Isc=4.75 A  Voc=0.6 V  Is=1e-6 A  Is2=0 A  Iph=7.34 A  Ir0=1000 W/m^2  ec=1.6  N2=2  Rs=5.1e-3 Ohm  Rp=Inf Ohm  TIPH1=0.65e-3 1/K  EG=1.12 eV  TXIS1=3  TXIS2=3  TRS1=0  TRP1=0  TFIXED=25 C  Tmeas=25 C  LocalVarLogging=[]
  Solar Cellc : elec_lib/Sources/Solar Cell  DialogController=NetworkEngine.DynNeDlgSource  SystemSampleTime=-1  prm=1  Isc=4.75 A  Voc=0.6 V  Is=1e-6 A  Is2=0 A  Iph=7.34 A  Ir0=1000 W/m^2  ec=1.6  N2=2  Rs=5.1e-3 Ohm  Rp=Inf Ohm  TIPH1=0.65e-3 1/K  EG=1.12 eV  TXIS1=3  TXIS2=3  TRS1=0  TRP1=0  TFIXED=25 C  Tmeas=25 C  LocalVarLogging=[]
  Solar Celld : elec_lib/Sources/Solar Cell  DialogController=NetworkEngine.DynNeDlgSource  SystemSampleTime=-1  prm=1  Isc=4.75 A  Voc=0.6 V  Is=1e-6 A  Is2=0 A  Iph=7.34 A  Ir0=1000 W/m^2  ec=1.6  N2=2  Rs=5.1e-3 Ohm  Rp=Inf Ohm  TIPH1=0.65e-3 1/K  EG=1.12 eV  TXIS1=3  TXIS2=3  TRS1=0  TRP1=0  TFIXED=25 C  Tmeas=25 C  LocalVarLogging=[]
  Solar Celle : elec_lib/Sources/Solar Cell  DialogController=NetworkEngine.DynNeDlgSource  SystemSampleTime=-1  prm=1  Isc=4.75 A  Voc=0.6 V  Is=1e-6 A  Is2=0 A  Iph=7.34 A  Ir0=1000 W/m^2  ec=1.6  N2=2  Rs=5.1e-3 Ohm  Rp=Inf Ohm  TIPH1=0.65e-3 1/K  EG=1.12 eV  TXIS1=3  TXIS2=3  TRS1=0  TRP1=0  TFIXED=25 C  Tmeas=25 C  LocalVarLogging=[]
  Solar Cellf : elec_lib/Sources/Solar Cell  DialogController=NetworkEngine.DynNeDlgSource  SystemSampleTime=-1  prm=1  Isc=4.75 A  Voc=0.6 V  Is=1e-6 A  Is2=0 A  Iph=7.34 A  Ir0=1000 W/m^2  ec=1.6  N2=2  Rs=5.1e-3 Ohm  Rp=Inf Ohm  TIPH1=0.65e-3 1/K  EG=1.12 eV  TXIS1=3  TXIS2=3  TRS1=0  TRP1=0  TFIXED=25 C  Tmeas=25 C  LocalVarLogging=[]
  Ir : PMIOPort  Port=1  Side=Left
  + : PMIOPort  Port=2  Side=Right
  - : PMIOPort  Port=3  Side=Left
  connections:
  Solar Celle/LConn1 -- Solar Cellf/LConn1 -- Ir/RConn1 -- Solar Celld/LConn1 -- Solar Cellc/LConn1 -- Solar Cella/LConn1 -- Solar Cellb/LConn1
  Solar Cella/RConn1 -- Solar Cellb/LConn2
  Solar Cellc/LConn2 -- Solar Cellb/RConn1
  Solar Celld/LConn2 -- Solar Cellc/RConn1
  Solar Celle/LConn2 -- Solar Celld/RConn1
  Solar Cellf/LConn2 -- Solar Celle/RConn1
  +/RConn1 -- Solar Cella/LConn2
  -/RConn1 -- Solar Cellf/RConn1

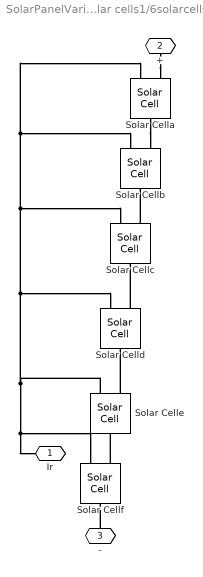
== system SolarPanelVarified/Solar module (72 cells)1/36 solarceel1/18 solar cells1/6solarcells1 ==
  Solar Cella : elec_lib/Sources/Solar Cell  DialogController=NetworkEngine.DynNeDlgSource  SystemSampleTime=-1  prm=1  Isc=4.75 A  Voc=0.6 V  Is=1e-6 A  Is2=0 A  Iph=7.34 A  Ir0=1000 W/m^2  ec=1.6  N2=2  Rs=5.1e-3 Ohm  Rp=Inf Ohm  TIPH1=0.65e-3 1/K  EG=1.12 eV  TXIS1=3  TXIS2=3  TRS1=0  TRP1=0  TFIXED=25 C  Tmeas=25 C  LocalVarLogging=[]
  Solar Cellb : elec_lib/Sources/Solar Cell  DialogController=NetworkEngine.DynNeDlgSource  SystemSampleTime=-1  prm=1  Isc=4.75 A  Voc=0.6 V  Is=1e-6 A  Is2=0 A  Iph=7.34 A  Ir0=1000 W/m^2  ec=1.6  N2=2  Rs=5.1e-3 Ohm  Rp=Inf Ohm  TIPH1=0.65e-3 1/K  EG=1.12 eV  TXIS1=3  TXIS2=3  TRS1=0  TRP1=0  TFIXED=25 C  Tmeas=25 C  LocalVarLogging=[]
  Solar Cellc : elec_lib/Sources/Solar Cell  DialogController=NetworkEngine.DynNeDlgSource  SystemSampleTime=-1  prm=1  Isc=4.75 A  Voc=0.6 V  Is=1e-6 A  Is2=0 A  Iph=7.34 A  Ir0=1000 W/m^2  ec=1.6  N2=2  Rs=5.1e-3 Ohm  Rp=Inf Ohm  TIPH1=0.65e-3 1/K  EG=1.12 eV  TXIS1=3  TXIS2=3  TRS1=0  TRP1=0  TFIXED=25 C  Tmeas=25 C  LocalVarLogging=[]
  Solar Celld : elec_lib/Sources/Solar Cell  DialogController=NetworkEngine.DynNeDlgSource  SystemSampleTime=-1  prm=1  Isc=4.75 A  Voc=0.6 V  Is=1e-6 A  Is2=0 A  Iph=7.34 A  Ir0=1000 W/m^2  ec=1.6  N2=2  Rs=5.1e-3 Ohm  Rp=Inf Ohm  TIPH1=0.65e-3 1/K  EG=1.12 eV  TXIS1=3  TXIS2=3  TRS1=0  TRP1=0  TFIXED=25 C  Tmeas=25 C  LocalVarLogging=[]
  Solar Celle : elec_lib/Sources/Solar Cell  DialogController=NetworkEngine.DynNeDlgSource  SystemSampleTime=-1  prm=1  Isc=4.75 A  Voc=0.6 V  Is=1e-6 A  Is2=0 A  Iph=7.34 A  Ir0=1000 W/m^2  ec=1.6  N2=2  Rs=5.1e-3 Ohm  Rp=Inf Ohm  TIPH1=0.65e-3 1/K  EG=1.12 eV  TXIS1=3  TXIS2=3  TRS1=0  TRP1=0  TFIXED=25 C  Tmeas=25 C  LocalVarLogging=[]
  Solar Cellf : elec_lib/Sources/Solar Cell  DialogController=NetworkEngine.DynNeDlgSource  SystemSampleTime=-1  prm=1  Isc=4.75 A  Voc=0.6 V  Is=1e-6 A  Is2=0 A  Iph=7.34 A  Ir0=1000 W/m^2  ec=1.6  N2=2  Rs=5.1e-3 Ohm  Rp=Inf Ohm  TIPH1=0.65e-3 1/K  EG=1.12 eV  TXIS1=3  TXIS2=3  TRS1=0  TRP1=0  TFIXED=25 C  Tmeas=25 C  LocalVarLogging=[]
  Ir : PMIOPort  Port=1  Side=Left
  + : PMIOPort  Port=2  Side=Right
  - : PMIOPort  Port=3  Side=Left
  connections:
  Solar Celle/LConn1 -- Solar Cellf/LConn1 -- Ir/RConn1 -- Solar Celld/LConn1 -- Solar Cellc/LConn1 -- Solar Cella/LConn1 -- Solar Cellb/LConn1
  Solar Cella/RConn1 -- Solar Cellb/LConn2
  Solar Cellc/LConn2 -- Solar Cellb/RConn1
  Solar Celld/LConn2 -- Solar Cellc/RConn1
  Solar Celle/LConn2 -- Solar Celld/RConn1
  Solar Cellf/LConn2 -- Solar Celle/RConn1
  +/RConn1 -- Solar Cella/LConn2
  -/RConn1 -- Solar Cellf/RConn1

== system SolarPanelVarified/Solar module (72 cells)1/36 solarceel1/18 solar cells1/6solarcells2 ==
  Solar Cella : elec_lib/Sources/Solar Cell  DialogController=NetworkEngine.DynNeDlgSource  SystemSampleTime=-1  prm=1  Isc=4.75 A  Voc=0.6 V  Is=1e-6 A  Is2=0 A  Iph=7.34 A  Ir0=1000 W/m^2  ec=1.6  N2=2  Rs=5.1e-3 Ohm  Rp=Inf Ohm  TIPH1=0.65e-3 1/K  EG=1.12 eV  TXIS1=3  TXIS2=3  TRS1=0  TRP1=0  TFIXED=25 C  Tmeas=25 C  LocalVarLogging=[]
  Solar Cellb : elec_lib/Sources/Solar Cell  DialogController=NetworkEngine.DynNeDlgSource  SystemSampleTime=-1  prm=1  Isc=4.75 A  Voc=0.6 V  Is=1e-6 A  Is2=0 A  Iph=7.34 A  Ir0=1000 W/m^2  ec=1.6  N2=2  Rs=5.1e-3 Ohm  Rp=Inf Ohm  TIPH1=0.65e-3 1/K  EG=1.12 eV  TXIS1=3  TXIS2=3  TRS1=0  TRP1=0  TFIXED=25 C  Tmeas=25 C  LocalVarLogging=[]
  Solar Cellc : elec_lib/Sources/Solar Cell  DialogController=NetworkEngine.DynNeDlgSource  SystemSampleTime=-1  prm=1  Isc=4.75 A  Voc=0.6 V  Is=1e-6 A  Is2=0 A  Iph=7.34 A  Ir0=1000 W/m^2  ec=1.6  N2=2  Rs=5.1e-3 Ohm  Rp=Inf Ohm  TIPH1=0.65e-3 1/K  EG=1.12 eV  TXIS1=3  TXIS2=3  TRS1=0  TRP1=0  TFIXED=25 C  Tmeas=25 C  LocalVarLogging=[]
  Solar Celld : elec_lib/Sources/Solar Cell  DialogController=NetworkEngine.DynNeDlgSource  SystemSampleTime=-1  prm=1  Isc=4.75 A  Voc=0.6 V  Is=1e-6 A  Is2=0 A  Iph=7.34 A  Ir0=1000 W/m^2  ec=1.6  N2=2  Rs=5.1e-3 Ohm  Rp=Inf Ohm  TIPH1=0.65e-3 1/K  EG=1.12 eV  TXIS1=3  TXIS2=3  TRS1=0  TRP1=0  TFIXED=25 C  Tmeas=25 C  LocalVarLogging=[]
  Solar Celle : elec_lib/Sources/Solar Cell  DialogController=NetworkEngine.DynNeDlgSource  SystemSampleTime=-1  prm=1  Isc=4.75 A  Voc=0.6 V  Is=1e-6 A  Is2=0 A  Iph=7.34 A  Ir0=1000 W/m^2  ec=1.6  N2=2  Rs=5.1e-3 Ohm  Rp=Inf Ohm  TIPH1=0.65e-3 1/K  EG=1.12 eV  TXIS1=3  TXIS2=3  TRS1=0  TRP1=0  TFIXED=25 C  Tmeas=25 C  LocalVarLogging=[]
  Solar Cellf : elec_lib/Sources/Solar Cell  DialogController=NetworkEngine.DynNeDlgSource  SystemSampleTime=-1  prm=1  Isc=4.75 A  Voc=0.6 V  Is=1e-6 A  Is2=0 A  Iph=7.34 A  Ir0=1000 W/m^2  ec=1.6  N2=2  Rs=5.1e-3 Ohm  Rp=Inf Ohm  TIPH1=0.65e-3 1/K  EG=1.12 eV  TXIS1=3  TXIS2=3  TRS1=0  TRP1=0  TFIXED=25 C  Tmeas=25 C  LocalVarLogging=[]
  Ir : PMIOPort  Port=1  Side=Left
  + : PMIOPort  Port=2  Side=Right
  - : PMIOPort  Port=3  Side=Left
  connections:
  Solar Celle/LConn1 -- Solar Cellf/LConn1 -- Ir/RConn1 -- Solar Celld/LConn1 -- Solar Cellc/LConn1 -- Solar Cella/LConn1 -- Solar Cellb/LConn1
  Solar Cella/RConn1 -- Solar Cellb/LConn2
  Solar Cellc/LConn2 -- Solar Cellb/RConn1
  Solar Celld/LConn2 -- Solar Cellc/RConn1
  Solar Celle/LConn2 -- Solar Celld/RConn1
  Solar Cellf/LConn2 -- Solar Celle/RConn1
  +/RConn1 -- Solar Cella/LConn2
  -/RConn1 -- Solar Cellf/RConn1
